simulink model "tanque_conico_planta_virtual_2015b_controlado"  (R2020a)
settings: Solver=ode45  StartTime=0.0  StopTime=4000  MaxStep=0.5  RelTol=1e-3
undefined symbols (not defined in the file or in its folder): h0_per, params, tanque_conico, tanque_conico_planta_virtual_params, theta0_per
settings Model: Creator=torres  LastModifiedBy=ean
settings OptimizationCC: LifeSpan=inf
settings DebuggingCC: SFExecutionAtInitializationDiag=none  ArithmeticOperatorsInVariantConditions=warning
settings SFSimCC: CustomCodeUndefinedFunction=UseInterfaceOnly
settings CodeAppCC: StateflowObjectComments=on

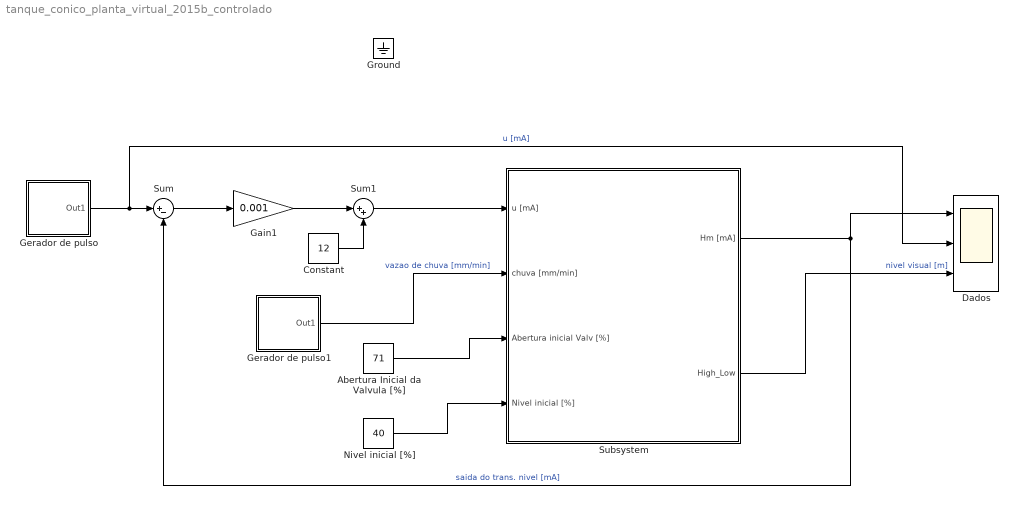
== system tanque_conico_planta_virtual_2015b_controlado ==
  Abertura Inicial da Valvula [%] : Constant  Value=71
  Constant : Constant  Value=12
  Dados : Scope  NumInputPorts=3
  Gain1 : Gain  Gain=0.001
  Gerador de pulso : Subsystem  mask{tpulso=500, deltat_pulso=100000, valor0_pulso=10.4, Apulso=3.2}
      mask prompts: tpulso "Tempo de inicio [s]"; deltat_pulso "Duração do pulso [s]"; valor0_pulso "Valor inicial"; Apulso "Amplitude do pulso (variação em relação ao valor inicial)"
  Gerador de pulso1 : Subsystem  mask{tpulso=3000, deltat_pulso=300, valor0_pulso=0, Apulso=100*0}
      mask prompts: tpulso "Tempo de inicio [s]"; deltat_pulso "Duração do pulso [s]"; valor0_pulso "Valor inicial"; Apulso "Amplitude do pulso (variação em relação ao valor inicial)"
  Nivel inicial [%] : Constant  Value=40
  Subsystem : Subsystem  InitFcn=|  StopFcn=tanque_conico_planta_virtual_params(0);
      | global params;
      | tanque_conico_planta_virtual_params(1);
      settings: OpenFcn=%
      mask Display: image('icon_sistema_tanque_com_chuva1.png')
  Sum : Sum  Inputs=|+-
  Sum1 : Sum  Inputs=|++
  Ground : Ground  IOType=siggen
  wires:
  Gerador de pulso1/1(Out1) -> Subsystem/2(chuva [mm/min])  "vazao de chuva [mm/min]"
  Subsystem/1(Hm [mA]) -> Dados/1, Sum/2  "saida do trans. nivel [mA]"
  Abertura Inicial da Valvula [%]/1 -> Subsystem/3(Abertura inicial Valv [%])
  Nivel inicial [%]/1 -> Subsystem/4(Nivel inicial [%])
  Subsystem/2(High_Low) -> Dados/3  "nivel visual [m]"
  Gain1/1 -> Sum1/1
  Sum1/1 -> Subsystem/1(u [mA])
  Constant/1 -> Sum1/2
  Sum/1 -> Gain1/1
  Gerador de pulso/1(Out1) -> Dados/2, Sum/1  "u [mA]"

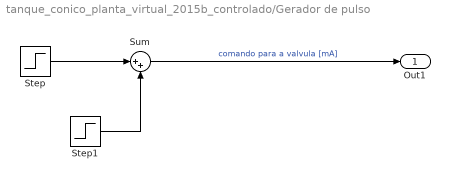
== system tanque_conico_planta_virtual_2015b_controlado/Gerador de pulso ==
  Step : Step  Time=tpulso  Before=valor0_pulso  After=valor0_pulso+Apulso  SampleTime=0
  Step1 : Step  Time=tpulso+deltat_pulso  After=-Apulso  SampleTime=0
  Sum : Sum  Inputs=|++
  Out1 : Outport
  wires:
  Step/1 -> Sum/1
  Step1/1 -> Sum/2
  Sum/1 -> Out1/1  "comando para a valvula [mA]"

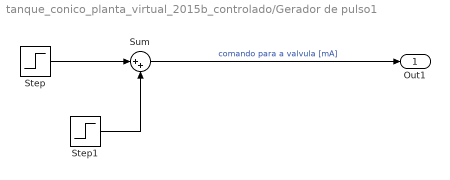
== system tanque_conico_planta_virtual_2015b_controlado/Gerador de pulso1 ==
  Step : Step  Time=tpulso  Before=valor0_pulso  After=valor0_pulso+Apulso  SampleTime=0
  Step1 : Step  Time=tpulso+deltat_pulso  After=-Apulso  SampleTime=0
  Sum : Sum  Inputs=|++
  Out1 : Outport
  wires:
  Step/1 -> Sum/1
  Step1/1 -> Sum/2
  Sum/1 -> Out1/1  "comando para a valvula [mA]"

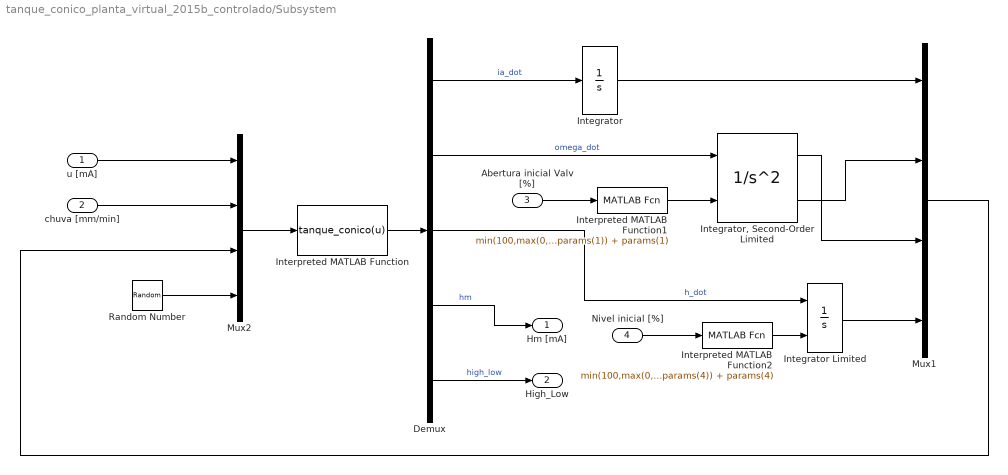
== system tanque_conico_planta_virtual_2015b_controlado/Subsystem ==
  u [mA] : Inport
  chuva [mm/min] : Inport  Port=2
  Abertura inicial Valv [%] : Inport  Port=3
  Nivel inicial [%] : Inport  Port=4
  Demux : Demux  Outputs=5
  Integrator : Integrator  ContinuousStateAttributes='x1'
  Integrator Limited : Integrator  InitialConditionSource=external  InitialCondition=params(4) + max(0,min(100,h0_per))/100*(params(3)-params(4))  LimitOutput=on  UpperSaturationLimit=params(3)  LowerSaturationLimit=params(4)  ContinuousStateAttributes='x4'
  "Integrator, Second-Order Limited" : SecondOrderIntegrator  ICSourceX=external  ICX=params(1) + max(0,min(100,theta0_per))/100*(params(2)-params(1))  LimitX=on  UpperLimitX=params(2)  LowerLimitX=params(1)  StateNameX='x3'  ICDXDT=0  StateNameDXDT='x2'  IgnoreStateLimitsAndResetForLinearization=on
  Interpreted MATLAB Function : MATLABFcn  MATLABFcn=tanque_conico(u)  OutputDimensions=5  OutputSignalType=real  Output1D=off
  Interpreted MATLAB Function1 : MATLABFcn  MATLABFcn=min(100,max(0,u))/100*(params(2)-params(1)) + params(1)
  Interpreted MATLAB Function2 : MATLABFcn  MATLABFcn=min(100,max(0,u))/100*(params(3)-params(4)) + params(4)
  Mux1 : Mux
  Mux2 : Mux
  Random Number : RandomNumber  Seed=floor(10*rand)  SampleTime=params(22)
  Hm [mA] : Outport
  High_Low : Outport  Port=2
  wires:
  Interpreted MATLAB Function/1 -> Demux/1
  Mux2/1 -> Interpreted MATLAB Function/1
  u [mA]/1 -> Mux2/1
  "Integrator, Second-Order Limited"/1 -> Mux1/3
  Demux/1 -> Integrator/1  "ia_dot"
  "Integrator, Second-Order Limited"/2 -> Mux1/2
  Abertura inicial Valv [%]/1 -> Interpreted MATLAB Function1/1
  Interpreted MATLAB Function2/1 -> Integrator Limited/2
  Mux1/1 -> Mux2/3
  Integrator/1 -> Mux1/1
  Random Number/1 -> Mux2/4
  chuva [mm/min]/1 -> Mux2/2
  Interpreted MATLAB Function1/1 -> "Integrator, Second-Order Limited"/2
  Nivel inicial [%]/1 -> Interpreted MATLAB Function2/1
  Demux/2 -> "Integrator, Second-Order Limited"/1  "omega_dot"
  Demux/3 -> Integrator Limited/1  "h_dot"
  Demux/4 -> Hm [mA]/1  "hm"
  Integrator Limited/1 -> Mux1/4
  Demux/5 -> High_Low/1  "high_low"
